simulink model "System_Modell"  (R2018a)
settings: Solver=FixedStepAuto  StartTime=0.0  StopTime=inf  FixedStep=1/f  RelTol=1e-3
values from neighbouring files (symbols this model uses):
  f = 10000    [System_Init.m]
(part 3 of 8)

== system System_Modell/ZP_Mananger/Schnittstelle_1/Send_Telegram ==
  status : Inport
  clock : Inport  Port=2
  lenS_1 : Inport  Port=3
  lenS_2 : Inport  Port=4
  Memory : Memory  InitialCondition=false
  Memory1 : Memory  InitialCondition=false
  Pulse : DiscretePulseGenerator  PulseType=Time based  Amplitude=true  Period=200/f  PulseWidth=30
  Send_Telegram : MATLAB Function  TreatAsAtomicUnit=on  SystemSampleTime=100/f
  Send_Telegram1 : MATLAB Function  TreatAsAtomicUnit=on  SystemSampleTime=100/f
  Tx_1_signal : Outport
  Tx_1_data : Outport  Port=2
  Tx_2_signal : Outport  Port=3
  Tx_2_data : Outport  Port=4
  wires:
  status/1 -> Send_Telegram1/1(status), Send_Telegram/1(status)
  clock/1 -> Send_Telegram1/2(clock), Send_Telegram/2(clock)
  Send_Telegram/1(Tx_1_signal) -> Tx_1_signal/1, Memory/1
  lenS_1/1 -> Send_Telegram/3(lenS_1)
  Memory/1 -> Send_Telegram/5(send_1_old)
  Send_Telegram/2(Tx_1_data) -> Tx_1_data/1
  Pulse/1 -> Send_Telegram1/4(impulse), Send_Telegram/4(impulse)
  Memory1/1 -> Send_Telegram1/5(send_2_old)
  Send_Telegram1/1(Tx_2_signal) -> Memory1/1, Tx_2_signal/1
  Send_Telegram1/2(Tx_2_data) -> Tx_2_data/1
  lenS_2/1 -> Send_Telegram1/3(lenS_2)

== system System_Modell/ZP_Mananger/GSM /ZP-Tabelle bearbeiten/add_new_ZP ==
  note: [n, Ax1, status, Ax2, status, Ax3, status]
  Adresse : Inport
  SkillRequest : Inport  Port=2
  last_Axis : Inport  Port=3
  n : Inport  Port=4
  Trigger : TriggerPort  VariantControl=Variant  PortDimensions=1
  add_new_ZP : MATLAB Function  TreatAsAtomicUnit=on
  send_SkillRequest : Outport
  Axis_remenber : Outport  Port=2
  n_remenber : Outport  Port=3
  wires:
  n/1 -> add_new_ZP/4(n)
  SkillRequest/1 -> add_new_ZP/2(SkillRequest)
  add_new_ZP/1(send_SkillRequest) -> send_SkillRequest/1
  last_Axis/1 -> add_new_ZP/3(SkillRequest_last)
  add_new_ZP/3(n_remember) -> n_remenber/1
  add_new_ZP/2(SkillRequest_remember) -> Axis_remenber/1
  Adresse/1 -> add_new_ZP/1(adr)

== matlab function System_Modell/Motor_1/MotionSM_1/MATLAB Function ==
  data: status input double size=1; excute_signal output boolean size=1; message_to_send output double size=2; data_received input double size=2; ZZP_wait data_store_memory size=1; AP data_store_memory; ZZP data_store_memory
%data_received / message_to_send = [cmd, ZZP]
%cmd:  1...setP, 2...getP, 3...excP

function [excute_signal, message_to_send] = message_analysis(status, data_received)

global ZZP_wait
global AP
global ZZP

excute_signal = false;

cmd = data_received(1);
message_to_send = [0, 0]';

switch cmd
    case 1      % setP
        excute_signal = false;
        if ((status >= 1) && (status <= 3))
            ZZP_wait = data_received(2);
            message_to_send = [2, ZZP_wait]';   % getP
        end
        
    case 3      % excP
        excute_signal = true;
        if ((ZZP == AP) && (status == 2) && (ZZP~=ZZP_wait))
            ZZP = ZZP_wait;
        end
end
end

== matlab function System_Modell/Motor_1/MotionSM_1/Motor/MATLAB Function ==
  settings: updateMethod=DISCRETE
  data: status_Motor output boolean size=1; Motor_control_signal input double size=1; parameter input double size=4; v input double size=1; a output double size=1; direction output double size=1; AP data_store_memory; ZZP data_store_memory
function [status_Motor, a, direction]= Motor(Motor_control_signal, parameter, v)

%delta_T = parameter(1);
a_max = abs(parameter(2));
v_max = abs(parameter(3));
s0 = parameter(4);
direction = 0;
a = 0;

s_a = 0.5 * v_max * v_max / a_max;
a_bremsen = 100000;     % 100 m/s^2

global AP
global ZZP

switch Motor_control_signal
    case {-1, 0}            %Error & Off
        if v > 0
            a = -a_bremsen;
            direction = 1;
        elseif v < 0
            a = a_bremsen;
            direction = -1;
        else
            a = 0;
            direction = 0;
        end
             
    case 1                  %Init
        if (AP > 0)
            direction = s0;
            if ((ZZP - AP) < (-s_a)) && (v > (-v_max))
                a = -a_max;
            elseif ((ZZP - AP) >= (-s_a)) && (ZZP < AP) && (v < 0)
                a = a_max;
            else
                a = 0;
            end
        else
            a = 0;
            AP = 0;
        end
        
    case 2                  %Stop
        if (v > 0)
            a = -a_max;
            direction = 1;
        elseif (v < 0)
            a = a_max;
            direction = -1;
        else
            a = 0;
            direction = 0;
        end
        
    case 3                  %run
        direction = s0;
        if (s0 > 0)   %forward
            %v_control(2) = s0;
            if ((ZZP - AP) > s_a) && (v < v_max)
                a = a_max;
            elseif ((ZZP - AP) <= s_a) && (ZZP > AP) && (v > 0)
                a = -a_max;
            else
                a = 0;
            end
        end
        if (s0 < 0)    %backward
            if ((ZZP - AP) < (-s_a)) && (v > (-v_max))
                a = -a_max;
            elseif ((ZZP - AP) >= (-s_a)) && (ZZP < AP) && (v < 0)
                a = a_max;
            else
                a = 0;
            end
        end
end
        
%status_Motor: false...Stopped, true...Running
if (a == 0) && (v == 0)
    status_Motor = false;
else
    status_Motor = true;
end

end

== stateflow chart System_Modell/Motor_1/MotionSM_1/Chart ==
  state Off
    entry: status=0;
  state Init
    entry: status=1; parameter=Par_1(delta_T);
  state On
    state Stop
      entry: status=2;
    state Run
      entry: status=3;
    (default) -> Stop
    Stop -> Run : [excute_signal==1 && ZZP~=AP && Motor_status == 0]
        | {parameter=Par(delta_T);}
    Run -> Stop : [ZZP==AP && ~Motor_status]
  state Error
    entry: status=-1;
  (default) -> Off
  Init -> Off [order 1] : [~EinAus]
  Off -> Init [order 2] : [EinAus && ~ NotAus]{parameter=[delta_T,0,0,0]';}
  Init -> Error [order 2] : [Motor_status==-1 || NotAus || ErrorSignal]
  Off -> Error [order 1] : [EinAus && (ErrorSignal || NotAus)]
  Error -> Off [order 1] : [~EinAus]
  On -> Off [order 1] : [~EinAus]
  Error -> Init [order 2] : [Richten]{parameter=[delta_T,0,0,0]';}
  Init -> On [order 3] : [AP==0]{parameter=[delta_T,0,0,0]';}
  On -> Error [order 2] : [Motor_status==-1 || NotAus || ErrorSignal]
  data: par function_output double size=4; delta_t function_input double size=1; par function_output double size=4; delta_t function_input double size=1; NotAus input boolean size=1; EinAus input boolean size=1; Richten input boolean size=1; ErrorSignal input boolean size=1; excute_signal input boolean size=1; Motor_status input boolean size=1; status output double size=1 =0; ZZP data_store_memory; ZZP_wait data_store_memory; parameter output double size=4; AP data_store_memory size=1; delta_T input double size=1
  function par = Par_1(delta_t):
    | function par = Par_1(delta_t)
    | 
    | global ZZP
    | global ZZP_wait
    | global AP
    | 
    | % delta_T = 10 s
    | ZZP = 0;
    | ZZP_wait = 0;
    | s0 = ZZP - AP;
    | a_max = 100;        % 1 m/s^2
    | v_max = 1;
    | %v_max = 0.5 * a_max * (delta_t - sqrt(delta_t*delta_t - 4*abs(s0)/a_max));   	% mm/s
    | 
    | par = [delta_t, a_max, v_max, s0]';
    | end
  function par = Par(delta_t):
    | function par = Par(delta_t)
    | 
    | global ZZP
    | global AP
    | 
    | s0 = ZZP - AP;
    | a_max = 1000;       % 1 m/s^2
    | v_max = 0.5 * a_max * (delta_t - sqrt(delta_t*delta_t - 4*abs(s0)/a_max));  % mm/s
    | 
    | par = [delta_t, a_max, v_max, s0]';
    | end

== matlab function System_Modell/Motor_1/MotionSM_1/Motor/MATLAB Function1 ==
  settings: updateMethod=DISCRETE
  data: V output; v input; direction input double size=1; AP data_store_memory; ZZP data_store_memory
function V = v_conrol(v, direction)

global AP
global ZZP

if direction > 0
    if ((v < 0) || (AP >= ZZP))
        V = 0;
    else
        V = v;
    end
elseif direction < 0
    if v > 0 || (AP <= ZZP)
        V = 0;
    else
        V = v;
    end
else
    V = 0;
end
end

== matlab function System_Modell/Motor_1/MotionSM_1/Motor/MATLAB Function2 ==
  settings: updateMethod=DISCRETE
  data: s input; s_old input; S output; direction input double size=1; AP data_store_memory; ZZP data_store_memory
function S = s_control(s, s_old, direction)

global AP
global ZZP

if direction > 0
    if (AP + s - s_old) < ZZP
        S = s;
        AP = AP + s - s_old;
    else
        S = s_old;
        AP = ZZP;
    end
elseif direction < 0
    if (AP + s - s_old) > ZZP
        S = s;
        AP = AP + s - s_old;
    else
        S = s_old;
        AP = ZZP;
    end
else
    S = s_old;
end

end

== stateflow chart System_Modell/Motor_1/CommSM_1/Status_Control ==
  state Init
    entry: 	status=1;
    send_AT_package=[Adresse, zeros(1,6)];
    send_signal=false;
    send_MotionSM=[0,0];
  state Aus
    entry: status=0;
  state Ein
    state State_Control [parallel]
      settings: executionOrder=1
      note: % Protokoll
          | % SummenTelegramm = [HDR, SDT, END]
          | %HDR: header, SDT: Summen-Daten-Telegramm, END: Ender
          |
          | % SDT = [SDT_7, SDT_1, SDT_2, SDT_3]
          | % SDT_i = [Da_i, De_i]
          | %Da: Data, De: Delay
          | %i...{1,2,3,7} %7...GSM, 1-3...CommSM1-3
          |
          | % Da_i = [sender, receiver, cmd, N, ZP, ZP_status]
          | %sender,receiver...{1,2,3,7,255} %255...Broadcast
          | %cmd: 1...addP, 2...getP, 3...setS, 4...getS
          | %ZP_status: 0...none, 1...wait, 2...active, 3...done, 4...error
          |
          | % Da_i = [sender, receiver, cmd, N, s , s _status]
          | %cmd: 5 ...negO
          | % s _status: 0...none, 1...negotiation, 2...excute, 3...done
      note: 问题
          | 如何检测下一个新的ZP
      state send_AT_2_GSM
        entry:	status=16;
        permission=true;
        send_AT_package=[Adresse, 7, 113, ZPT(N,1:3), 0];
        %AT=[CommSM, GSM, setS, n, ZP, done];
        send_signal=true;
      state Free
        entry:	status=2;
      state Arrival
        entry:	status=15;
        ZPT(N,3)=3;
      state check_ZPT
        entry:	status=3;
        ZPT(N,3)=2;	      % status='active'
      state wait_arrival
        entry: status=14
      state send_Status_activ
        entry:	status=4;
        permission = true;
        send_AT_package = [Adresse, 7, 113, ZPT(N,1:3), 0];
        % AT=[CommSM, GSM, setS, n, ZP, activ];
        send_signal = true;
      state check_ZP
        entry: 	status=5;
        s=checkZP(ZZP_old, Adresse, N);
        % s-range: [0, 100], ZZP_old: ZZP for last loop
      state MotionSM
        entry:	status=13;
        send_MotionSM=[3, ZZPT(Adresse,2)];	%excute ZZP
        a = ZPT(N,2); b = ZZPT(Adresse,2);
      state send_nego_1
        entry: 	status=6;
        permission = true;
        send_AT_package=[Adresse, 255, 115, ZPT(N,1), s, 1, 0];
        % AT=[CommSM, Broadcast, negO, n, s, nego];
        send_signal=true;
      state Nego_wait
        entry: 	status=7;
      state send_excu
        entry:	status=12;
        permission = true;
        send_AT_package = [Adresse, 255, 115, ZPT(N,1), ZZPT(Adresse, 4), 2, 0];
        %AT=[CommSM, Broadcast, negO, n, s, excu];
        send_signal = true;
      state Wait_excution
        entry:	status=11;
        send_MotionSM=[1, ZZPT(Adresse,2)]; %set ZZP
      state s_Compair
        entry: 	status=8;
        s_new=s_compair(Adresse);
      state status_excution
        entry: 	status=10;
        ZZPT(Adresse,4)=2; %excu
      state ZZP_new
        entry:	status=9;
        ZZPT(Adresse,3)=s_new;
        ZZPT(Adresse,2)=AP+(ZPT(N,2)-AP)*(s_new/100);
      (default) -> Free
      send_AT_2_GSM -> Free : [send_done]{send_signal=false; permission = false;}
      Free -> check_ZPT : % status ='wait' && MotionSM kein Fehler
          | [N>0 && ZPT(N,3)==1 && status_MotionSM>=1]{send_signal = false;}
      (junction 77) -> send_AT_2_GSM : [~permission]
      Arrival -> (junction 77)
      (junction 121) -> (junction 77)
      wait_arrival -> Arrival : % ZP == ZZP -> wait until ZP == AP
          | [isequal([ZPT(N,2), status_MotionSM],[AP, 2])]
          | {ZZPT=zeros(3,4);}
      check_ZPT -> send_Status_activ : [ZPT(N,3)==2 && ~permission]
      MotionSM -> wait_arrival [order 2] : % ZP == ZZP -> ZP will be arrived & no next ZP -> end
          | [status_MotionSM==3 && a==b && isempty(find(ZPT(:,3)==1,1))]
          | {send_MotionSM=zeros(1,2)}
      (junction 116) -> (junction 99)
      (junction 148) -> (junction 116)
      send_Status_activ -> (junction 99) : [send_done]{send_signal = false; permission = false;}
      (junction 99) -> check_ZP
      MotionSM -> (junction 116) [order 1] : % ZP~=ZZP -> ZP will not be arrived -> negotiate again
          | [status_MotionSM==3 && a~=b]
          | {ZZP_old = ZZPT(Adresse,2); ZZPT = zeros(3,4);}
      MotionSM -> (junction 148) [order 3] : [false]
          | % ZP = ZZP -> ZP will be arrived -> new ZP wait to negotiate -> loop
          | %[status_MotionSM==3 && a==b && ~isempty(find(ZPT(:,3)==1,1))]
          | %{ZZP_old = ZZPT(Adresse,2); ZZPT = zeros(3,4)}
      check_ZP -> send_nego_1 : [~permission]
      (junction 146) -> MotionSM : % Motor stoped
          | [status_MotionSM==2]
      (junction 216) -> (junction 146) : % all axis excuteable && received ZZP from MotionSM
          | [isequal(ZZPT(1:3,4),[2;2;2]) && isequal(data_from_MotionSM(1:2),[2,ZZPT(Adresse,2)])]
          | {ZZP_old=0;}
      send_nego_1 -> Nego_wait : [send_done]{s=0; send_signal=false; permission = false;}
      send_excu -> (junction 216) : [send_done]{send_signal=false; permission = false;}
      Nego_wait -> (junction 121) [order 1] : % ZP = AP, ZP schon erreicht
          | [ZPT(N,3)==3]
      Nego_wait -> (junction 134) [order 2] : % ZP~=AP, ZP "activ"
          | [ZPT(N,3)==2]
      Wait_excution -> send_excu : [~permission]
      (junction 134) -> s_Compair : % ob ZZPT komplett erfüllt
          | [isequal(ZZPT(1:3,1),[1,1,1]')]
      status_excution -> Wait_excution : [status_MotionSM>=2]  % 2 or 3
      s_Compair -> (junction 79)
      (junction 66) -> status_excution : {s_new=0;}
      (junction 79) -> (junction 66) [order 2] : [s_new>=ZZPT(Adresse,3)]
      (junction 79) -> ZZP_new [order 1] : [s_new<ZZPT(Adresse,3)]
      ZZP_new -> (junction 66)
    state Send [parallel]
      settings: executionOrder=2
      state wait
      state send
        entry: permission = true;
        send_AT_package = [Adresse, 7, 2, ZPT(n-1,1:3),0];
        send_signal = true;
      (default) -> wait
      wait -> (junction 181) : % Requirement to respond GSM
          | [respond]
      send -> wait : % send done
          | [send_done]{respond = false;send_signal = false; permission = false;}
      (junction 181) -> send : % permission to use send_port
          | [~permission]
  state Error
    entry: status=-1;
  (default) -> Aus
  Aus -> Init : [EinAus && ~NotAus && ~ErrorSignal]
  Init -> Aus [order 2] : [~EinAus]
  Init -> Error [order 3] : [NotAus]
  Error -> Aus [order 1] : [~EinAus]
  Ein -> Aus [order 1] : [~EinAus]
  Error -> Init [order 2] : [Richten && ~NotAus && ~ErrorSignal]
  Init -> Ein [order 1] : [status_Schnittstelle==4]{send_signal=false;}
  Ein -> Error [order 2] : [NotAus]
  data: zzp_old function_input double size=1; S function_output; adress function_input double size=1; N_ function_input; S_new function_output double size=1; nr function_input double size=1; Adresse input double size=1; status_Schnittstelle input double size=1; n input; N input; NotAus input boolean size=1; EinAus input boolean size=1; Richten input boolean size=1; ErrorSignal input boolean size=1; send_done input; status output double size=1; send_signal output boolean size=1 =false; send_AT_package output double size=[1,7] =zeros(1,7); status_MotionSM input double size=1; data_from_MotionSM input double size=[1,2]; ZPT data_store_memory; ZZPT data_store_memory; AP data_store_memory; s local double size=1 =0; s_new local double size=1 =0; send_MotionSM output double size=[1,2] =zeros(1,2); ZZP_old local double size=1 =0; permission local boolean size=1 =false; respond data_store_memory; a local; b local
  function S = checkZP(zzp_old, adress, N_):
    | %ZPT = [10x3], [ZP_Nr., ZP, status]
    | %status: {0...none, 1...wait, 2...active, 3...done, 4...error}
    | 
    | %ZZPT(CommSM_i,:) = [ZP-Nr., ZZP, s%, status]
    | %status: {0...none, 1...negotiation, 2...excution, 3...done}
    | 
    | function S = checkZP(zzp_old, adress, N_)
    | %1. prüfen, ob ZP unter begrenzte Bedienung erreichbar ist
    |         %Ja     --> ZZP = ZP
    |         %Nein   --> neuen ZZP erzeugen
    | %2. neu ausgerechnete ZZP in der ZZP Tabelle einschreiben
    |  
    | global AP
    | global ZPT
    | global ZZPT
    | 
    | a_max = 1000;   % mm/s^2
    | v_max = 1000;   % mm/s
    | d_T = 10;    % s
    | 
    | s_max = a_max*d_T*d_T/4;
    | if zzp_old <= 0             %last ZZP to arrive. After the Motor is started, ZZP_old = ZZP, ZZPT = zeros(3,4);
    |     s0 = ZPT(N_,2) - AP;     %ZP - AP
    | else
    |     s0 = ZPT(N_,2) - zzp_old;    %excist last ZZP
    | end
    | 
    | if abs(s0) <= s_max
    |     S = 100;                    % 100% erreichbar
    | elseif abs(s0) > 0 && abs(s0) < 100
    |     S = abs(100*s_max/s0);      % s% s: [0, 100]
    |     S = fix(1000*S)/1000;       % Genauigkeit = 10000*0.001%=0.1 mm
    | else
    |     S = 0;                      % ZP = AP, Achse keine Bewegung
    | end
    | 
    | %ZZP-Tabelle erfüllen
    | if zzp_old <= 0
    |     ZZP_new = AP + s0*S/100;        %neue ZZP in der ZZP-Tabelle einschreiben
    | else
    |     ZZP_new = zzp_old+s0*S/100;
    | end
    | 
    | if S == 0
    |     ZPT(N_,3) = 3;
    | else
    |     ZZPT(adress,:) = [ZPT(N_,1), ZZP_new, S, 1];
    | end
    | 
    | end
  function S_new = s_compair(nr):
    | function S_new = s_compair(nr)
    | 
    | global ZZPT
    | 
    | s_ = ZZPT(:,3);
    | 
    | S_new = s_(nr);          % CommSM_me
    | 
    | for i = 1:3                         % s==0 --> s=100
    |     if i ~= nr && s_(i)== 0
    |         s_(i) = 100;
    |     end
    | end
    | 
    | s_min = min(s_);
    | if S_new > s_min
    |     S_new = s_min;
    | end
    | 
    | end

== matlab function System_Modell/Motor_1/CommSM_1/MATLAB Function ==
  data: status input; n input; N input; signal input boolean size=1; package input double size=[1,7]; ZPT data_store_memory; ZZPT data_store_memory; respond data_store_memory
%Protokoll
%SummenTelegramm = [HDR, SDT, END]
	%HDR: header,	SDT: Summen-Daten-Telegramm,    END: Ender

%SDT = [SDT_7, SDT_1, SDT_2, SDT_3]
%SDT_i = [Da_i, De_i]
	%Da: Data, De: Delay
	%i...{1,2,3,7}	%7...GSM, 1-3...CommSM1-3

%Da_i = [sender, receiver, cmd, N, ZP, ZP_status]
	%sender,receiver...{1,2,3,7,255}	%255...Broadcast
	%cmd: 111...addP, 112...getP, 113...setS, 114...getS
	%ZP_status: 0...none, 1...wait, 2...active, 3...done, 4...error

%Da_i = [sender, receiver, cmd, N, s, s_status]
	%cmd: 115...negO
	%s_status: 0...none, 1...negotiation, 2...excute, 3...done


% Hier werden nur die Befehlen, die ZPT oder ZZPT ändern möchte, werden behandelt.
function receive_AT(status, n, N, signal, package)

% n - the first free row in ZPT to add new ZP
% N - the line of currently handled ZP in ZPT

global ZPT
global ZZPT
global respond              % respond requirement, to let "send_AT" know, that it should answer the GSM

if (signal && (status >= 2))
    switch package(1)       % from GSM
        case 7
            switch package(3)
                case 111                    % cmd == 'add Position'
                    if (isempty(find(ZPT(:,1)==package(4),1)) && (n >= 1) && (n <= 10))
                        ZPT(n,:) = package(4:6)'; %[n, ZP, status='wait']
                        respond = true;
                    end
            end
            
        case {2,3}          % from CommSM_2 or CommSM_3
            switch package(3)
                case 115                    % negotiation
                    if ((N > 0) && (package(4) == ZPT(N,1)))
                        switch package(6)
                            case 1      % nego
                                if status == 7
                                    ZZPT(package(1),:) = [package(4), 0, package(5:6)];     % [n, ZP, s%, status='nego']
                                end
                            case 2      % excu
                                if ((status == 12) && (ZZPT(package(1),4) == 1))
                                    ZZPT(package(1),4) = package(6);                        % [n, ZP, s%, status='excu']
                                end
                        end
                    end
            end
    end
end

end

== matlab function System_Modell/Motor_2/CommSM_1/MATLAB Function ==
  data: status input; n input; N input; signal input boolean size=1; package input double size=[1,7]; ZPT data_store_memory; ZZPT data_store_memory; respond data_store_memory
%Protokoll
%SummenTelegramm = [HDR, SDT, END]
	%HDR: header,	SDT: Summen-Daten-Telegramm,    END: Ender

%SDT = [SDT_7, SDT_1, SDT_2, SDT_3]
%SDT_i = [Da_i, De_i]
	%Da: Data, De: Delay
	%i...{1,2,3,7}	%7...GSM, 1-3...CommSM1-3

%Da_i = [sender, receiver, cmd, N, ZP, ZP_status]
	%sender,receiver...{1,2,3,7,255}	%255...Broadcast
	%cmd: 111...addP, 112...getP, 113...setS, 114...getS
	%ZP_status: 0...none, 1...wait, 2...active, 3...done, 4...error

%Da_i = [sender, receiver, cmd, N, s, s_status]
	%cmd: 115...negO
	%s_status: 0...none, 1...negotiation, 2...excute, 3...done


% Hier werden nur die Befehlen, die ZPT oder ZZPT ändern möchte, werden behandelt.
function receive_AT(status, n, N, signal, package)

% n - the first free row in ZPT to add new ZP
% N - the line of currently handled ZP in ZPT

global ZPT
global ZZPT
global respond              % respond requirement, to let "send_AT" know, that it should answer the GSM

if (signal && (status >= 2))
    switch package(1)       % from GSM
        case 7
            switch package(3)
                case 111                    % cmd == 'add Position'
                    if (isempty(find(ZPT(:,1)==package(4),1)) && (n >= 1) && (n <= 10))
                        ZPT(n,:) = package(4:6)'; %[n, ZP, status='wait']
                        respond = true;
                    end
            end
            
        case {2,3}          % from CommSM_2 or CommSM_3
            switch package(3)
                case 115                    % negotiation
                    if ((N > 0) && (package(4) == ZPT(N,1)))
                        switch package(6)
                            case 1      % nego
                                if status == 7
                                    ZZPT(package(1),:) = [package(4), 0, package(5:6)];     % [n, ZP, s%, status='nego']
                                end
                            case 2      % excu
                                if ((status == 12) && (ZZPT(package(1),4) == 1))
                                    ZZPT(package(1),4) = package(6);                        % [n, ZP, s%, status='excu']
                                end
                        end
                    end
            end
    end
end

end

== matlab function System_Modell/Motor_1/CommSM_1/MATLAB Function2 ==
  data: n output; N output; ZPT data_store_memory
% n - the first free row in ZPT to add new ZP
% N - the line of currently handled ZP in ZPT

function [n,N] = counter

global ZPT

if ~isempty(find(ZPT(:,1)==0,1))
    n = min(find(ZPT(:,1)==0,1));
else
    n = 11;
end

done = find(ZPT(:,3)==3,1);
active = find(ZPT(:,3)==2,1);
wait = find(ZPT(:,3)==1,1);
if isempty(done)
    if ZPT(1,1) >= 1
        N = 1;
    else
        N = 0;
    end
else
	if ~isempty(active)
        N = max(active);
    elseif ~isempty(wait)
        N = min(wait);
    else
        N = max(done);
end

end

== matlab function System_Modell/Motor_2/CommSM_1/MATLAB Function2 ==
  data: n output; N output; ZPT data_store_memory
% n - the first free row in ZPT to add new ZP
% N - the line of currently handled ZP in ZPT

function [n,N] = counter

global ZPT

if ~isempty(find(ZPT(:,1)==0,1))
    n = min(find(ZPT(:,1)==0,1));
else
    n = 11;
end

done = find(ZPT(:,3)==3,1);
active = find(ZPT(:,3)==2,1);
wait = find(ZPT(:,3)==1,1);
if isempty(done)
    if ZPT(1,1) >= 1
        N = 1;
    else
        N = 0;
    end
else
	if ~isempty(active)
        N = max(active);
    elseif ~isempty(wait)
        N = min(wait);
    else
        N = max(done);
end

end

== matlab function System_Modell/Motor_1/Schnittstelle_0/Add_to_Send_Buffer ==
  data: Send_Buffer_1 data_store_memory; Send_Buffer_2 data_store_memory; Address data_store_memory; status input; lenS_1 input; lenS_2 input; to_send_signal input; to_send_package input; Address_1 data_store_memory; Address_2 data_store_memory; Handshake_1 data_store_memory; Handshake_2 data_store_memory; Filter data_store_memory; De_1 data_store_memory; De_2 data_store_memory; De_sum_1 data_store_memory; De_sum_2 data_store_memory
% Name: add_to_Send_Buffer
% Funktionalitäten
% Handshake-Message einfügen, wenn Status==1
% Delay-caculation-Message einfügen, wenn Status==2
% Sum-Delay-caculation-Message einfügen, wemm Status==3
% Nachrichten, die der Host senden möchte, einfügen, wenn Status==4

function add_to_Send_Buffer(status, lenS_1, lenS_2, to_send_signal, to_send_package)

global Send_Buffer_1
global Send_Buffer_2
global Address
global Address_1
global Address_2
global Handshake_1
global Handshake_2
global Filter
global De_1
global De_2
global De_sum_1
global De_sum_2

switch status
    case -2                         % Error Signal einrichten
        Filter(1,7) = 1;
    case 1                          % Handshake
        if((Filter(1,1) == 0) && ~Handshake_1)              % 103 not sent yet || Handshake_1 not finish yet
            check_1 = check_X(103, Address, Send_Buffer_1);          % check if there is a 103-Message in Send_Buffer_1
            if ~check_1
                Send_Buffer_1(lenS_1:lenS_1+7) = [Address, 0, 103, zeros(1,4), 102];
                Filter(1,1) = 1;                            % to remember, if 103 ist sent
            end
        end
        if((Filter(1,2) == 0) && ~Handshake_2)
            check_2 = check_X(103, Address, Send_Buffer_2);
            if ~check_2
                Send_Buffer_2(lenS_2:lenS_2+7) = [Address, 0, 103, zeros(1,4), 102];
                Filter(1,2) = 1;
            end
        end

        
    case 2                          % Delay time caculation
        if((Filter(1,3) == 0 ) && (De_1 <= 0))              % 105 not sent || De_1 not caculated yet
            check_1 = check_X(105, Address, Send_Buffer_1);
            if ~check_1
                Send_Buffer_1(lenS_1:lenS_1+7) = [Address, Address_2, 105, zeros(1,4), 102];
                Filter(1,3) = 1;
            end
        end
        if((Filter(1,4) == 0 ) && (De_2 <= 0))
            check_2 = check_X(105, Address, Send_Buffer_2);
            if ~check_2
                Send_Buffer_2(lenS_2:lenS_2+7) = [Address, Address_1, 105, zeros(1,4), 102];
                Filter(1,4) = 1;
            end
        end
        
    case 3                          % Sum_Delay caculation
        if((Filter(1,5) == 0 ) && (De_sum_1 <= 0))          % 107 not sent || De_sum_1 not caculated yet
            check_1 = check_X(107, Address, Send_Buffer_1);
            if ~check_1
                Send_Buffer_1(lenS_1:lenS_1+7) = [Address, Address, 107, zeros(1,4), 102];
                Filter(1,5) = 1;
            end
        end
        if((Filter(1,6) == 0 ) && (De_sum_2 <= 0))
            check_2 = check_X(107, Address, Send_Buffer_2);
            if ~check_2
                Send_Buffer_2(lenS_2:lenS_2+7) = [Address, Address, 107, zeros(1,4), 102];
                Filter(1,6) = 1;
            end
        end
        
    case 4                          % normal communication
        if to_send_signal
            check_1 = check_Y(to_send_package, Send_Buffer_1);
            check_2 = check_Y(to_send_package, Send_Buffer_2);
            if ~check_1
                Send_Buffer_1(lenS_1:lenS_1+7) = [to_send_package, 102];
            end
            if ~check_2
                Send_Buffer_2(lenS_2:lenS_2+7) = [to_send_package, 102];
            end
        end
end

end

function y = check_X(CMD, adr, Data)          % y: boolean; x: double, [1x100];

x = find(Data==CMD);
y = ~isempty(x);
if y
    y = y && (Data(1,x(1)-2) == adr);
end

end

function y = check_Y(data, Data)          % y: boolean; data: double, [1x6];

x = find(Data==data(3));        % CMD
y = ~isempty(x);
if y
    for i=1:length(x)
        if(isequal(Data(x(i)-2:x(i)+3),data(1:6)))
            y = true;
            break
        else
            y = false;
        end
    end
end

end

== matlab function System_Modell/Motor_1/Schnittstelle_0/Global_Var_Length ==
  data: len_Send_Buffer_1 output double size=1; len_Send_Buffer_2 output double size=1; len_Recv_Buffer output double size=1; len_Filter output double size=1; Send_Buffer_1 data_store_memory; Send_Buffer_2 data_store_memory; Recv_Buffer data_store_memory; Filter data_store_memory
% genutzte Länge der globale Variablen berechnen

function [len_Send_Buffer_1, len_Send_Buffer_2, len_Recv_Buffer, len_Filter] = Length
global Send_Buffer_1
global Send_Buffer_2
global Recv_Buffer
global Filter

a1 = find(Send_Buffer_1==102,1);
len_Send_Buffer_1 = a1(1);
a2 = find(Send_Buffer_2==102,1);
len_Send_Buffer_2 = a2(1);

len_Recv_Buffer = min(find(Recv_Buffer==0,150))-1;
len_Filter = min(find(Filter(2:20)==0,150));

end

== matlab function System_Modell/Motor_1/Schnittstelle_0/Recv_1 ==
  data: status input double size=1; clock input double size=1; lenS_1 input; lenS_2 input; lenR input; Rx_1_signal input boolean size=1; Rx_1_data input double size=[1 100]; recv_signal_1 output boolean; recv_package_1 output double size=[1 98]; Send_Buffer_1 data_store_memory; Send_Buffer_2 data_store_memory; T_send_1 data_store_memory; T_recv_1 data_store_memory; De_1 data_store_memory; De_sum_1 data_store_memory; Address data_store_memory; Recv_Buffer data_store_memory; Address_2 data_store_memory; Address_1 data_store_memory; De_sum_2 data_store_memory; Handshake_1 data_store_memory; De_2 data_store_memory; Handshake_2 data_store_memory; T_recv_2 data_store_memory; T_send_2 data_store_memory
% Name: Rx_1

% -------------------------------------------------------------------------------------
% Funktionalitäten:
% Im Init-Prozess
%   1. Handshake durch zu führen
%       103...Handshake ask --> 104 in Send_Buffer_2 additieren
%       104...Handshake answer --> Handshake success
%   2. Delay-Zeit berechnen
%       105...Delay begin --> 106 in Send_Buffer_2 additieren
%       106...Delay end --> Delay_Zeit berechnen
%   3. Sum-Delay-Zeit berechnen
%       107, Receiver = meine Addresse --> Sum_Delay_Zeit berechnen
%       107, Receiver ~= meine Addresse --> Daten in Send_Buffer_1 additieren
% Im normalen Prozess
%   4. Receiver = meine Addresse --> in Recv_Buffer additieren
%   5. Receiver = 255 --> Broadcast --> in Recv_Buffer && Send_Buffer_1 additieren
%   6. Receiver ~= meine Addresse --> in Send_Buffer_1 additieren

% -------------------------------------------------------------------------------------
% Input && Output
% status - status of 'Schnittstelle'
% clock - simulation time
% lenS_1/len_2/lenR - meaningful length of Send_Buffer_1/Send_Buffer_2/Recv_Buffer
% Rx_1_data - from Rx_1 received data
% recv_package_1 - data to send to chart or store in Send_Buffer_1
    % in Init-process, recv_package_1 need to be sent to chart
    % in normal-process, recv_package_1 need to garther all 'to be transmmited' datablock, and store in Send_Buffer_1

function [recv_signal_1, recv_package_1] = Rx_1(status, clock,lenS_1, lenS_2, lenR, Rx_1_signal, Rx_1_data)

global Send_Buffer_1
global Send_Buffer_2
global T_send_1
global T_recv_1
global De_1
%global De_2
global De_sum_1
global Address
global Address_1
%global Address_2
global Recv_Buffer
global Handshake_1

recv_signal_1 = false;
recv_package_1 = zeros(1,98);       % one datablock = [1x7]

lenr = 1;                           % path to write data into recv_package_1

if Rx_1_signal
    a = find(Rx_1_data==102,1);
    len = a(1);
    if ~isempty(len)
        mod_ = mod(len-2,7);
        len_ = ceil((len - 2) / 7);                                 % Round toward positive infinity
    end
    
	if ((mod_ == 0) && (len_ >= 1))                             % package contains at least one datablock
        switch status
            case 1                                              % Handshake
                for i=1:len_
                    switch Rx_1_data(7*i-3)                          % Da.cmd
                        case 103                                % Handshake ask --> send answer
                            check = check_X(104, Address, Send_Buffer_2);
                            if ((Rx_1_data(7*i-5) ~= 0) && (Rx_1_data(7*i-4) == 0) && ~Handshake_1 && ~check)
                                Address_1 = Rx_1_data(7*i-5);
                                Send_Buffer_2(lenS_2:lenS_2+7) = [Address, Address_1, 104, zeros(1,4), 102];
                            end
                        case 104                                % Handshake answer --> Handshake success --> no more send
                            if ((Rx_1_data(7*i-5) ~= 0) && (Rx_1_data(7*i-4) == Address) && ~Handshake_1)
                                Address_1 = Rx_1_data(7*i-5);        % Address of the Host in the Direction_1
                                recv_package_1(lenr:lenr+6) = Rx_1_data(7*i-5:7*i+1);    % [_,_,104,_,_,_,_] = [1x7]
                                lenr = lenr + 7;
                                recv_signal_1 = true;
                            end
                    end
                end

            case 2                                              % Delay_Time_Caculation
                for j=1:len_
                    switch Rx_1_data(7*j-3)                          % Da.cmd
                        case 103                                % Handshake ask --> send answer
                            check = check_X(104, Address, Send_Buffer_2);
                            if ((Rx_1_data(7*j-5) ~= 0) && (Rx_1_data(7*j-4) == 0) && ~Handshake_1 && ~check)
                                Address_1 = Rx_1_data(7*j-5);
                                Send_Buffer_2(lenS_2:lenS_2+7) = [Address, Address_1, 104, zeros(1,4), 102];
                            end
                        case 105                                % Delay ask --> send answer
                            check = check_X(106, Address, Send_Buffer_2);
                            if (isequal(Rx_1_data(7*j-5:7*j-4),[Address_1, Address]) && Handshake_1 && ~check) % check Sender & Receiver
                                Send_Buffer_2(lenS_2:lenS_2+7) = [Address, Address_1, 106, zeros(1,4), 102];
                            end
                        case 106                                % Delay answer --> caculate the time --> no more send
                            if ((isequal(Rx_1_data(7*j-5:7*j-3),[Address_1, Address, 106])) && (De_1 <= 0) && (T_send_1 > 0))
                                T_recv_1 = clock;
                                De_1 = T_recv_1 - T_send_1;
                                T_send_1 = 0;
                                T_recv_1 = 0;
                            end
                    end
                end

            case 3                                              % Sum_Delay_Caculation
                for h=1:len_
                    switch Rx_1_data(7*h-3)
                        case 103                                % Handshake ask --> send answer
                            check = check_X(104, Address, Send_Buffer_2);
                            if ((Rx_1_data(7*h-5) ~= 0) && (Rx_1_data(7*h-4) == 0) && ~Handshake_1 && ~check)
                                Address_1 = Rx_1_data(7*h-5);
                                Send_Buffer_2(lenS_2:lenS_2+7) = [Address, Address_1, 104, zeros(1,4), 102];
                            end
                        case 105                                % Delay ask --> send answer
                            check = check_X(106, Address, Send_Buffer_2);
                            if (isequal(Rx_1_data(7*h-5:7*h-4),[Address_1, Address]) && Handshake_1 && ~check) % check Sender & Receiver
                                Send_Buffer_2(lenS_2:lenS_2+7) = [Address, 0, 106, zeros(1,4), 102];
                            end   
                        case 107
                            if (isequal(Rx_1_data(7*h-5:7*h-4),[Address, Address]) && (De_sum_1 <= De_1) && (T_send_1 > 0))                   % Sum_Delay --> caculate the time --> no more send
                                T_recv_1 = clock;
                                De_sum_1 = T_recv_1 - T_send_1;
                                T_send_1 = 0;
                                T_recv_1 = 0;
                            elseif ((isequal(Rx_1_data(7*h-5),Rx_1_data(7*h-4))) && (Rx_1_data(7*h-5) ~= Address))
                                check = check_Y(Rx_1_data(7*h-5:7*h), recv_package_1) || check_Y(Rx_1_data(7*h-5:7*h), Send_Buffer_1);
                                if ~check
                                    recv_package_1(lenr:lenr+6) = Rx_1_data(7*h-5:7*h+1)';
                                    lenr = lenr + 7;
                                end
                            end
                    end
                end
                Send_Buffer_1(lenS_1:lenS_1+lenr-1) = [recv_package_1(1:lenr-1),102];           % 前提：lenS更新速度比当前更新快

            case 4                                               % normal communication between all Hosts
                for k=1:len_
                    switch Rx_1_data(7*k-3)
                        case 103                                % Handshake ask --> send answer
                            check = check_X(104, Address, Send_Buffer_2);
                            if ((Rx_1_data(7*k-5) ~= 0) && (Rx_1_data(7*k-4) == 0) && ~Handshake_1 && ~check)
                                Address_1 = Rx_1_data(7*k-5);
                                Send_Buffer_2(lenS_2:lenS_2+7) = [Address, Address_1, 104, zeros(1,4), 102];
                            end
                        case 105                                % Delay ask --> send answer
                            check = check_X(106, Address, Send_Buffer_2);
                            if (isequal(Rx_1_data(7*k-5:7*k-4),[Address_1, Address]) && Handshake_1 && ~check) % check Sender & Receiver
                                Send_Buffer_2(lenS_2:lenS_2+7) = [Address, 0, 106, zeros(1,4), 102];
                            end
                        case 107
                            if ((isequal(Rx_1_data(7*k-5),Rx_1_data(7*k-4))) && (Rx_1_data(7*k-5) ~= Address))
                                check = check_Y(Rx_1_data(7*k-5:7*k), recv_package_1) || check_Y(Rx_1_data(7*k-5:7*k), Send_Buffer_1);
                                if ~check
                                    recv_package_1(lenr:lenr+6) = Rx_1_data(7*k-5:7*k+1)';
                                    lenr = lenr + 7;
                                end
                            end
                        otherwise
                            if ((Rx_1_data(7*k-5) ~= Address) && (Rx_1_data(7*k-4) == Address))   % Datablock sent to me --> store in Recv_Buffer
                                check = check_Y(Rx_1_data(7*k-5:7*k), Recv_Buffer');
                                if ~check
                                    Recv_Buffer(lenR+1,:) = Rx_1_data(7*k-5:7*k+1);
                                end
                            elseif ((Rx_1_data(7*k-5) ~=Address) && (Rx_1_data(7*k-4) == 255))    % Datablock is as a Broadcast --> store in Recv_Buffer && Send_Buffer_1
                                check = check_Y(Rx_1_data(7*k-5:7*k), Recv_Buffer');
                                if ~check
                                    Recv_Buffer(lenR+1,:) = Rx_1_data(7*k-5:7*k+1);
                                end
                                check = check_Y(Rx_1_data(7*k-5:7*k), recv_package_1) || check_Y(Rx_1_data(7*k-5:7*k), Send_Buffer_1);
                                if ~check
                                    recv_package_1(lenr:lenr+6) = Rx_1_data(7*k-5:7*k+1)';
                                    lenr = lenr + 7;
                                end
                            elseif ((Rx_1_data(7*k-4) ~= Address) && (Rx_1_data(7*k-4) ~= 255))   % Datablock not sent to me --> to transmmit --> store in Send_Buffer_1
                                check = check_Y(Rx_1_data(7*k-5:7*k), recv_package_1) || check_Y(Rx_1_data(7*k-5:7*k), Send_Buffer_1);
                                if ~check
                                    recv_package_1(lenr:lenr+6) = Rx_1_data(7*k-5:7*k+1)';
                                    lenr = lenr + 7;
                                end
                            end
                    end
                end
                Send_Buffer_1(lenS_1:lenS_1+lenr-1) = [recv_package_1(1:lenr-1),102];
        end
	elseif mod_ ~= 0
        fprintf("Eroor: Package length not avalueable!");
	end
end

end

% check_X: to check if Data contains a Datablock with CMD and adr
function y = check_X(CMD, adr, Data)          % y: boolean; x: double, [1x100];

x = find(Data==CMD);
y = (~isempty(x));

if y
    y = y && (Data(1,x(1)-2) == adr);
end

end

% check_Y: to check if Data contains data
function y = check_Y(data, Data)          % y: boolean; data: double, [1x6];

x = find(Data==data(3));
y = (~isempty(x));
if y
    for i=1:length(x)
        if(isequal(Data(x(i)-2:x(i)+3),data))
            y = true;
            break
        else
            y = false;
        end
    end
end

end
